simulink model "sim_lab2"  (R2020a)
settings: Solver=VariableStepAuto  StartTime=0.0  StopTime=60.0  RelTol=1e-3
values from neighbouring files (symbols this model uses):
  beta = 0.1    [lab2.m]
  kp = 1/mod_Hf    (= 1.64437172321)    [lab2.m]
  Ti = 4/wc    (= 13.3779264214)    [lab2.m]
  Ts = 0.1    [lab2.m]
undefined symbols (not defined in the file or in its folder): tau_d
settings Model: Creator=magor  LastModifiedBy=magor

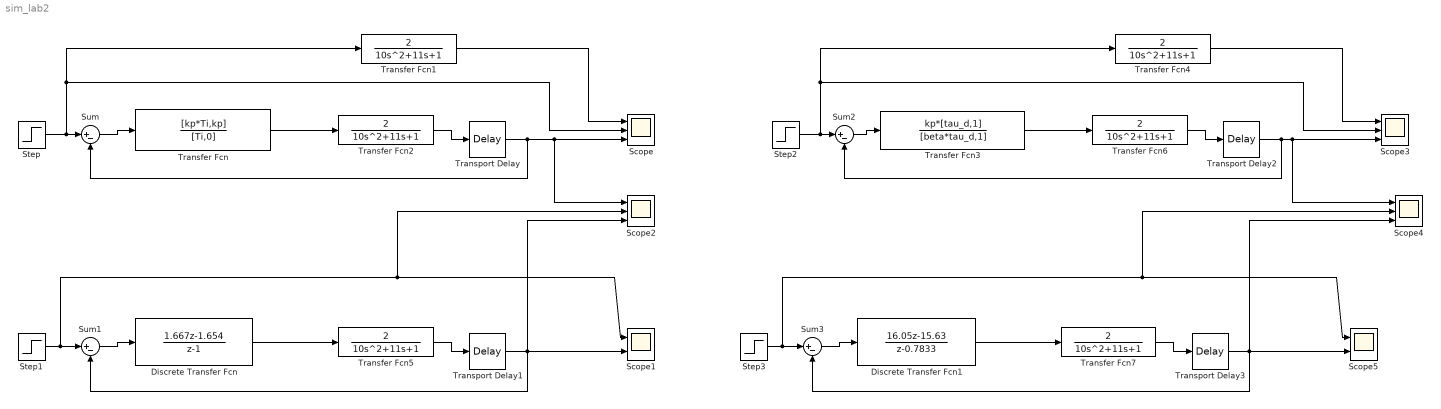
== system sim_lab2 ==
  Discrete Transfer Fcn : DiscreteTransferFcn  Numerator=[1.667, -1.654]  Denominator=[1 -1]  SampleTime=Ts
  Discrete Transfer Fcn1 : DiscreteTransferFcn  Numerator=[16.05, -15.63]  Denominator=[1 -0.7833]  SampleTime=Ts
  Scope{,2..4} (4 alike) : Scope  NumInputPorts=3
  Scope1 : Scope  NumInputPorts=2
  Scope5 : Scope  NumInputPorts=2
  Step{,1..3} (4 alike) : Step  Time=0  SampleTime=0
  Sum{,1..3} (4 alike) : Sum  Inputs=|+-
  Transfer Fcn : TransferFcn  Numerator=[kp*Ti,kp]  Denominator=[Ti,0]
  Transfer Fcn{1..2,4..7} (6 alike) : TransferFcn  Numerator=[2]  Denominator=[10 11 1]
  Transfer Fcn3 : TransferFcn  Numerator=kp*[tau_d,1]  Denominator=[beta*tau_d,1]
  Transport Delay{,1..3} (4 alike) : TransportDelay
  wires:
  Step/1 -> Transfer Fcn1/1, Scope/2, Sum/1
  Sum/1 -> Transfer Fcn/1
  Transfer Fcn1/1 -> Scope/1
  Transfer Fcn/1 -> Transfer Fcn2/1
  Transfer Fcn2/1 -> Transport Delay/1
  Transport Delay/1 -> Scope2/1, Scope/3, Sum/2
  Transfer Fcn5/1 -> Transport Delay1/1
  Transport Delay1/1 -> Scope2/3, Scope1/2, Sum1/2
  Sum1/1 -> Discrete Transfer Fcn/1
  Step1/1 -> Scope2/2, Scope1/1, Sum1/1
  Discrete Transfer Fcn/1 -> Transfer Fcn5/1
  Transfer Fcn6/1 -> Transport Delay2/1
  Transport Delay2/1 -> Scope4/1, Scope3/3, Sum2/2
  Transfer Fcn3/1 -> Transfer Fcn6/1
  Transfer Fcn4/1 -> Scope3/1
  Sum2/1 -> Transfer Fcn3/1
  Step2/1 -> Transfer Fcn4/1, Scope3/2, Sum2/1
  Step3/1 -> Scope4/2, Scope5/1, Sum3/1
  Transport Delay3/1 -> Scope4/3, Scope5/2, Sum3/2
  Transfer Fcn7/1 -> Transport Delay3/1
  Sum3/1 -> Discrete Transfer Fcn1/1
  Discrete Transfer Fcn1/1 -> Transfer Fcn7/1
